simulink model "RBDmodel"  (R2023a)
settings: Solver=ode15s  StartTime=0.0  StopTime=4  FixedStep=0.0001  RelTol=1e-3  AbsTol=1e-3  EnableMultiTasking=on
model workspace (MAT data in the model file):
  C_Gimbal = 0.5
  C_IAP = 0.01
  IAP_Pa = 0
  K_Gimbal = 0
  K_IAP = 200
  LeftAbdominalMuscleForce = 0
  LeftBackMuscleForce = 0
  LeftTransverse1MuscleForce = 0
  LeftTransverse2MuscleForce = 0
  Moment_AR = 0
  Moment_FE = 7.5
  Moment_LB = 0
  RightAbdominalMuscleForce = 0
  RightBackMuscleForce = 0
  RightTransverse1MuscleForce = 0
  RightTransverse2MuscleForce = 0
  a = 1
  b = 1
  muscle_color = [0 0 1]
  muscle_radius = 1
libraries: checkpacklib x3, simulink x1
(part 2 of 2)

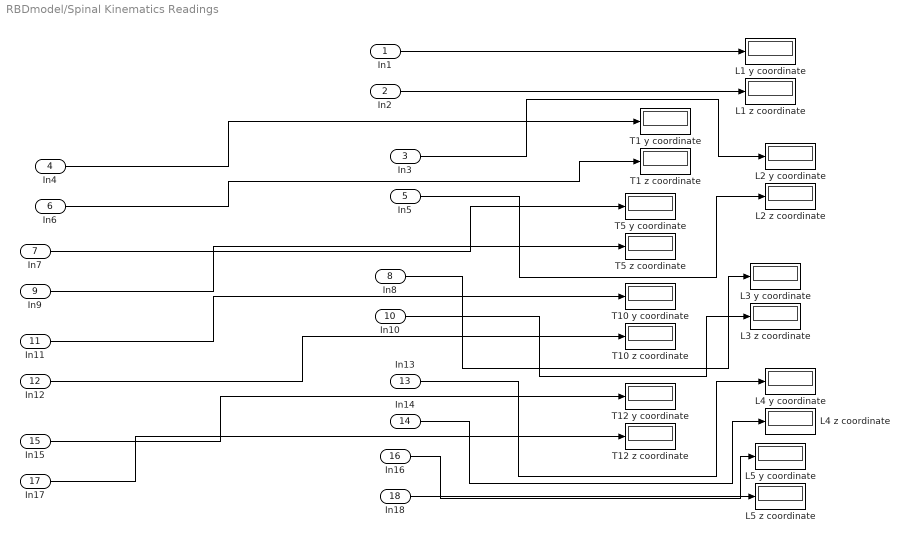
== system RBDmodel/Spinal Kinematics Readings ==
  In1 : Inport
  In2 : Inport  Port=2
  In3 : Inport  Port=3
  In4 : Inport  Port=4
  In5 : Inport  Port=5
  In6 : Inport  Port=6
  In7 : Inport  Port=7
  In8 : Inport  Port=8
  In9 : Inport  Port=9
  In10 : Inport  Port=10
  In11 : Inport  Port=11
  In12 : Inport  Port=12
  In13 : Inport  Port=13
  In14 : Inport  Port=14
  In15 : Inport  Port=15
  In16 : Inport  Port=16
  In17 : Inport  Port=17
  In18 : Inport  Port=18
  L1 y coordinate : Display
  L1 z coordinate : Display
  L2 y coordinate : Display
  L2 z coordinate : Display
  L3 y coordinate : Display
  L3 z coordinate : Display
  L4 y coordinate : Display
  L4 z coordinate : Display
  L5 y coordinate : Display
  L5 z coordinate : Display
  T1 y coordinate : Display
  T1 z coordinate : Display
  T10 y coordinate : Display
  T10 z coordinate : Display
  T12 y coordinate : Display
  T12 z coordinate : Display
  T5 y coordinate : Display
  T5 z coordinate : Display
  wires:
  In2/1 -> L1 z coordinate/1
  In7/1 -> T5 y coordinate/1
  In13/1 -> L4 y coordinate/1
  In10/1 -> L3 z coordinate/1
  In18/1 -> L5 z coordinate/1
  In6/1 -> T1 z coordinate/1
  In3/1 -> L2 y coordinate/1
  In11/1 -> T10 y coordinate/1
  In9/1 -> T5 z coordinate/1
  In1/1 -> L1 y coordinate/1
  In5/1 -> L2 z coordinate/1
  In14/1 -> L4 z coordinate/1
  In15/1 -> T12 y coordinate/1
  In4/1 -> T1 y coordinate/1
  In12/1 -> T10 z coordinate/1
  In8/1 -> L3 y coordinate/1
  In17/1 -> T12 z coordinate/1
  In16/1 -> L5 y coordinate/1

== matlab function RBDmodel/Muscle force inputs/Sum of Square of Forces ==
  data: F1 input; SumofSquareofForces output; F2 input; F3 input; F4 input; F5 input; F6 input; F7 input; F8 input; IAP input
function SumofSquareofForces = fcn(F1,F2,F3,F4,F5,F6,F7,F8,IAP)

SumofSquareofForces = F1^2 + F2^2 + F3^2 + F4^2 + F5^2 + F6^2 +F7^2 + F8^2 + IAP^2;
